simulink model "CSWI"  (Simulink 7.8)
settings: Solver=ode3  StartTime=0.0  StopTime=t_sim  FixedStep=1/6400  MaxStep=0.001  MinStep=0.000005  RelTol=1e-3
StopFcn:
  | ComtradeWrite5( RDRE1_UIabc, RDRE1_ANames, RDRE1_Dsignals, RDRE1_DNames, RDRE1_ADCscale, RDRE1_PromtFile, RDRE1_NumFile, RDRE1_FileFormat, RDRE1_TestNum);
  | clear RDRE1_UIabc RDRE1_ANames RDRE1_Dsignals RDRE1_DNames RDRE1_ADCscale  RDRE1_PromtFile RDRE1_NumFile RDRE1_FileFormat RDRE1_TestNum
values from neighbouring files (symbols this model uses):
  BlkTmms1 = 700    [CSWI_SG1.m]    (also in CSWI_SG2.m = 650; CSWI_SG3.m; CSWI_SG4.m; CSWI_SG5.m)
  BlkTmms2 = 800    [CSWI_SG1.m]    (also in CSWI_SG2.m = 750; CSWI_SG3.m; CSWI_SG4.m; CSWI_SG5.m)
  ClsTmms1 = 250    [CSWI_SG1.m]    (also in CSWI_SG2.m = 200; CSWI_SG3.m; CSWI_SG4.m; CSWI_SG5.m)
  ClsTmms2 = 170    [CSWI_SG1.m]    (also in CSWI_SG2.m = 100; CSWI_SG3.m; CSWI_SG4.m; CSWI_SG5.m)
  ClsTmms3 = 60    [CSWI_SG1.m]    (also in CSWI_SG2.m = 30; CSWI_SG3.m; CSWI_SG4.m; CSWI_SG5.m)
  ClsTmms4 = 10    [CSWI_SG1.m]    (also in CSWI_SG2.m = 20; CSWI_SG3.m; CSWI_SG4.m; CSWI_SG5.m)
  FailTmms = 350    [CSWI_SG1.m]    (also in CSWI_SG2.m = 300; CSWI_SG3.m; CSWI_SG4.m; CSWI_SG5.m)
  FctMod1 = 1    [CSWI_SG1.m]    (also in CSWI_SG2.m; CSWI_SG3.m; CSWI_SG4.m; CSWI_SG5.m)
  FctMod2 = 1    [CSWI_SG1.m]    (also in CSWI_SG2.m; CSWI_SG3.m; CSWI_SG4.m = 0; CSWI_SG5.m)
  FctMod3 = 1    [CSWI_SG1.m]    (also in CSWI_SG2.m; CSWI_SG3.m; CSWI_SG4.m; CSWI_SG5.m = 0)
  Num_SG = 1    [CSWI_generate_tests.m]
  OpnTmms1 = 300    [CSWI_SG1.m]    (also in CSWI_SG2.m = 250; CSWI_SG3.m; CSWI_SG4.m; CSWI_SG5.m)
  OpnTmms2 = 200    [CSWI_SG1.m]    (also in CSWI_SG2.m = 150; CSWI_SG3.m; CSWI_SG4.m; CSWI_SG5.m)
  OpnTmms3 = 30    [CSWI_SG1.m]    (also in CSWI_SG2.m = 90; CSWI_SG3.m = 90; CSWI_SG4.m; CSWI_SG5.m)
  test_dc = 'Ïðîâåðêà îòñóòñòâèÿ ôîðìèðîâàíèÿ ñèãíàëîâ "Âêë." ïðè ôîðìèðîâàíèè ñèãíàëà  "Îòêë. îò ÄÓ"'    [CSWI_generate_tests.m]
undefined symbols (not defined in the file or in its folder): sigbuilder_block, Test_num
libraries: powerlib_extras x21
(part 3 of 3)

== system CSWI/CSWI/Положение блок-контактов/BlkTmms1/ON Delay ==
  IN : Inport
  DELAY : Inport  Port=2
  Enable : EnablePort  PropagateVarSize=During execution
  Constant2 : Constant  Value=-Ts
  Constant3 : Constant  Value=Ts
  Discrete Edge Detector : powerlib_extras/Discrete  Control Blocks/Discrete Edge Detector  model=Rising  ic=ic  Ts=Ts
  Logical Operator1 : Logic
  Relational Operator : RelationalOperator  OutDataTypeStr=boolean  InputSameDT=on
  Sum1 : Sum  Inputs=+-  SaturateOnIntegerOverflow=on  InputSameDT=on  OutDataTypeStr=Inherit: Same as first input
  Switch : Switch  Threshold=0.5  SaturateOnIntegerOverflow=on  InputSameDT=on
  Unit Delay : UnitDelay  SampleTime=Ts
  OUT : Outport
  wires:
  Unit Delay/1 -> Switch/3
  Sum1/1 -> Unit Delay/1, Relational Operator/2
  Switch/1 -> Sum1/1
  Constant3/1 -> Sum1/2
  Relational Operator/1 -> Logical Operator1/2
  IN/1 -> Discrete Edge Detector/1, Logical Operator1/1
  Logical Operator1/1 -> OUT/1
  DELAY/1 -> Switch/1
  Discrete Edge Detector/1 -> Switch/2
  Constant2/1 -> Relational Operator/1

== system CSWI/CSWI/Положение блок-контактов/BlkTmms2/OFF Delay ==
  IN : Inport
  DELAY : Inport  Port=2
  Enable : EnablePort  PropagateVarSize=During execution
  Constant2 : Constant  Value=-Ts
  Constant3 : Constant  Value=Ts
  Discrete Edge Detector : powerlib_extras/Discrete  Control Blocks/Discrete Edge Detector  model=Falling  ic=ic  Ts=Ts
  Logical Operator1 : Logic
  Logical Operator2 : Logic  Operator=NOT
  Logical Operator3 : Logic  Operator=NOT
  Relational Operator : RelationalOperator  OutDataTypeStr=boolean  InputSameDT=on
  Sum1 : Sum  Inputs=+-  SaturateOnIntegerOverflow=on  InputSameDT=on  OutDataTypeStr=Inherit: Same as first input
  Switch : Switch  Threshold=0.5  SaturateOnIntegerOverflow=on  InputSameDT=on
  Unit Delay : UnitDelay  SampleTime=Ts
  OUT : Outport
  wires:
  Unit Delay/1 -> Switch/3
  Sum1/1 -> Relational Operator/2, Unit Delay/1
  Switch/1 -> Sum1/1
  Constant3/1 -> Sum1/2
  Relational Operator/1 -> Logical Operator1/2
  IN/1 -> Discrete Edge Detector/1, Logical Operator2/1
  Logical Operator1/1 -> Logical Operator3/1
  DELAY/1 -> Switch/1
  Discrete Edge Detector/1 -> Switch/2
  Constant2/1 -> Relational Operator/1
  Logical Operator2/1 -> Logical Operator1/1
  Logical Operator3/1 -> OUT/1

== system CSWI/CSWI/Положение блок-контактов/BlkTmms2/ON Delay ==
  IN : Inport
  DELAY : Inport  Port=2
  Enable : EnablePort  PropagateVarSize=During execution
  Constant2 : Constant  Value=-Ts
  Constant3 : Constant  Value=Ts
  Discrete Edge Detector : powerlib_extras/Discrete  Control Blocks/Discrete Edge Detector  model=Rising  ic=ic  Ts=Ts
  Logical Operator1 : Logic
  Relational Operator : RelationalOperator  OutDataTypeStr=boolean  InputSameDT=on
  Sum1 : Sum  Inputs=+-  SaturateOnIntegerOverflow=on  InputSameDT=on  OutDataTypeStr=Inherit: Same as first input
  Switch : Switch  Threshold=0.5  SaturateOnIntegerOverflow=on  InputSameDT=on
  Unit Delay : UnitDelay  SampleTime=Ts
  OUT : Outport
  wires:
  Unit Delay/1 -> Switch/3
  Sum1/1 -> Unit Delay/1, Relational Operator/2
  Switch/1 -> Sum1/1
  Constant3/1 -> Sum1/2
  Relational Operator/1 -> Logical Operator1/2
  IN/1 -> Discrete Edge Detector/1, Logical Operator1/1
  Logical Operator1/1 -> OUT/1
  DELAY/1 -> Switch/1
  Discrete Edge Detector/1 -> Switch/2
  Constant2/1 -> Relational Operator/1

== system CSWI/CSWI/Положение блок-контактов/BlkTmms3/OFF Delay ==
  IN : Inport
  DELAY : Inport  Port=2
  Enable : EnablePort  PropagateVarSize=During execution
  Constant2 : Constant  Value=-Ts
  Constant3 : Constant  Value=Ts
  Discrete Edge Detector : powerlib_extras/Discrete  Control Blocks/Discrete Edge Detector  model=Falling  ic=ic  Ts=Ts
  Logical Operator1 : Logic
  Logical Operator2 : Logic  Operator=NOT
  Logical Operator3 : Logic  Operator=NOT
  Relational Operator : RelationalOperator  OutDataTypeStr=boolean  InputSameDT=on
  Sum1 : Sum  Inputs=+-  SaturateOnIntegerOverflow=on  InputSameDT=on  OutDataTypeStr=Inherit: Same as first input
  Switch : Switch  Threshold=0.5  SaturateOnIntegerOverflow=on  InputSameDT=on
  Unit Delay : UnitDelay  SampleTime=Ts
  OUT : Outport
  wires:
  Unit Delay/1 -> Switch/3
  Sum1/1 -> Relational Operator/2, Unit Delay/1
  Switch/1 -> Sum1/1
  Constant3/1 -> Sum1/2
  Relational Operator/1 -> Logical Operator1/2
  IN/1 -> Discrete Edge Detector/1, Logical Operator2/1
  Logical Operator1/1 -> Logical Operator3/1
  DELAY/1 -> Switch/1
  Discrete Edge Detector/1 -> Switch/2
  Constant2/1 -> Relational Operator/1
  Logical Operator2/1 -> Logical Operator1/1
  Logical Operator3/1 -> OUT/1

== system CSWI/CSWI/Положение блок-контактов/BlkTmms3/ON Delay ==
  IN : Inport
  DELAY : Inport  Port=2
  Enable : EnablePort  PropagateVarSize=During execution
  Constant2 : Constant  Value=-Ts
  Constant3 : Constant  Value=Ts
  Discrete Edge Detector : powerlib_extras/Discrete  Control Blocks/Discrete Edge Detector  model=Rising  ic=ic  Ts=Ts
  Logical Operator1 : Logic
  Relational Operator : RelationalOperator  OutDataTypeStr=boolean  InputSameDT=on
  Sum1 : Sum  Inputs=+-  SaturateOnIntegerOverflow=on  InputSameDT=on  OutDataTypeStr=Inherit: Same as first input
  Switch : Switch  Threshold=0.5  SaturateOnIntegerOverflow=on  InputSameDT=on
  Unit Delay : UnitDelay  SampleTime=Ts
  OUT : Outport
  wires:
  Unit Delay/1 -> Switch/3
  Sum1/1 -> Unit Delay/1, Relational Operator/2
  Switch/1 -> Sum1/1
  Constant3/1 -> Sum1/2
  Relational Operator/1 -> Logical Operator1/2
  IN/1 -> Discrete Edge Detector/1, Logical Operator1/1
  Logical Operator1/1 -> OUT/1
  DELAY/1 -> Switch/1
  Discrete Edge Detector/1 -> Switch/2
  Constant2/1 -> Relational Operator/1

== system CSWI/CSWI/РФК и Аварийное отключение/Discrete Bistable7/RESET Priority ==
  S : Inport
  R : Inport  Port=2
  Enable : EnablePort  PropagateVarSize=During execution
  IC = ic : UnitDelay  X0=ic  SampleTime=Ts
  Logical Operator : Logic  Operator=OR
  Logical Operator1 : Logic  Operator=NOT  Inputs=1
  Logical Operator2 : Logic
  Logical Operator3 : Logic  Operator=NOT  Inputs=1
  Q : Outport
  !Q : Outport  Port=2
  wires:
  Logical Operator2/1 -> Q/1, Logical Operator3/1, IC = ic/1
  Logical Operator1/1 -> Logical Operator2/2
  R/1 -> Logical Operator1/1
  Logical Operator/1 -> Logical Operator2/1
  IC = ic/1 -> Logical Operator/2
  Logical Operator3/1 -> !Q/1
  S/1 -> Logical Operator/1

== system CSWI/CSWI/РФК и Аварийное отключение/Discrete Bistable7/SET  Priority ==
  S : Inport
  R : Inport  Port=2
  Enable : EnablePort  PropagateVarSize=During execution
  IC = ic : UnitDelay  X0=ic  SampleTime=Ts
  Logical Operator : Logic  Operator=OR
  Logical Operator1 : Logic  Operator=NOT  Inputs=1
  Logical Operator2 : Logic
  Logical Operator3 : Logic  Operator=NOT  Inputs=1
  Q : Outport
  !Q : Outport  Port=2
  wires:
  S/1 -> Logical Operator/1
  Logical Operator3/1 -> !Q/1
  Logical Operator/1 -> IC = ic/1, Logical Operator3/1, Q/1
  R/1 -> Logical Operator1/1
  Logical Operator1/1 -> Logical Operator2/1
  IC = ic/1 -> Logical Operator2/2
  Logical Operator2/1 -> Logical Operator/2

== system CSWI/CSWI/Блок включения/ClsTmms2/Edge_Detector/NEGATIVE Edge ==
  IN : Inport
  IN previous : Inport  Port=2
  Enable : EnablePort  PropagateVarSize=During execution
  Relational Operator1 : RelationalOperator  Operator=>  InputSameDT=on
  OUT : Outport
  wires:
  IN/1 -> Relational Operator1/2
  IN previous/1 -> Relational Operator1/1
  Relational Operator1/1 -> OUT/1

== system CSWI/CSWI/Блок включения/ClsTmms2/Edge_Detector/POSITIVE Edge ==
  IN : Inport
  IN previous : Inport  Port=2
  Enable : EnablePort  PropagateVarSize=During execution
  Relational Operator1 : RelationalOperator  Operator=>  InputSameDT=on
  OUT : Outport
  wires:
  IN/1 -> Relational Operator1/1
  IN previous/1 -> Relational Operator1/2
  Relational Operator1/1 -> OUT/1

== system CSWI/CSWI/Блок отключения/OpnTmms2/Edge_Detector/NEGATIVE Edge ==
  IN : Inport
  IN previous : Inport  Port=2
  Enable : EnablePort  PropagateVarSize=During execution
  Relational Operator1 : RelationalOperator  Operator=>  InputSameDT=on
  OUT : Outport
  wires:
  IN/1 -> Relational Operator1/2
  IN previous/1 -> Relational Operator1/1
  Relational Operator1/1 -> OUT/1

== system CSWI/CSWI/Блок отключения/OpnTmms2/Edge_Detector/POSITIVE Edge ==
  IN : Inport
  IN previous : Inport  Port=2
  Enable : EnablePort  PropagateVarSize=During execution
  Relational Operator1 : RelationalOperator  Operator=>  InputSameDT=on
  OUT : Outport
  wires:
  IN/1 -> Relational Operator1/1
  IN previous/1 -> Relational Operator1/2
  Relational Operator1/1 -> OUT/1

== matlab function DREGOUT1/MATLAB Function ==
  data: u input double; SG_1 output double; SG_2 output double; SG_3 output double; SG_4 output double; SG_5 output double; SG_6 output double
% function [SG_1,SG_2,SG_3,SG_4]= fcn(u)
function [SG_1,SG_2,SG_3,SG_4,SG_5,SG_6]= fcn(u)
%#codegen
SG_1=0; SG_2=0; SG_3=0; SG_4=0; SG_5=0; SG_6=0;


if u ==2;
    SG_1=1;
elseif u ==3;
    SG_2=1;
elseif u ==4;
    SG_1=1; SG_2=1;
elseif u ==5;
    SG_3=1;
elseif u ==6;
    SG_1=1; SG_3=1;
elseif u ==7;
    SG_2=1; SG_3=1;
elseif u ==8;
    SG_1=1; SG_2=1; SG_3=1;
elseif u ==9;
    SG_4=1;
elseif u ==10;
    SG_1=1; SG_4=1;
elseif u ==11;
    SG_2=1; SG_4=1;
elseif u ==12;
    SG_1=1; SG_2=1; SG_4=1;
elseif u ==13;
    SG_3=1; SG_4=1;
elseif u ==14;
    SG_1=1; SG_3=1; SG_4=1;
elseif u ==15;
    SG_2=1; SG_3=1; SG_4=1;
elseif u ==16;
    SG_1=1; SG_2=1; SG_3=1; SG_4=1;
elseif u ==17;
    SG_5=1;
    
elseif u ==18;
       SG_5=1; SG_1=1;  
elseif u ==19;
       SG_5=1; SG_2=1;     
elseif u ==20;
       SG_5=1; SG_2=1; SG_1=1; 
elseif u ==21;
       SG_5=1; SG_3=1; 
elseif u ==22;
       SG_5=1; SG_3=1; SG_1=1;
elseif u ==23;
       SG_5=1; SG_3=1; SG_2=1;
elseif u ==24;
       SG_5=1; SG_3=1; SG_2=1; SG_1=1;
elseif u ==25;
       SG_5=1; SG_4=1;
elseif u ==26;
       SG_5=1; SG_4=1; SG_1=1;
elseif u ==27;
       SG_5=1; SG_4=1; SG_2=1;
elseif u ==28;
       SG_5=1; SG_4=1; SG_2=1; SG_1=1;
elseif u ==29;
       SG_5=1; SG_4=1; SG_3=1;    
elseif u ==30;
       SG_5=1; SG_4=1; SG_3=1; SG_1=1;
elseif u ==31;
       SG_5=1; SG_4=1; SG_3=1; SG_2=1;
elseif u ==32;
       SG_5=1; SG_4=1; SG_3=1; SG_2=1; SG_1=1;
elseif u ==33;
       SG_6=1;
elseif u ==34;
       SG_6=1; SG_1=1;
elseif u ==35;
       SG_6=1; SG_2=1;
elseif u ==36;
       SG_6=1; SG_2=1; SG_1=1;
elseif u ==37;
       SG_6=1; SG_3=1;
elseif u ==38;
       SG_6=1; SG_3=1; SG_1=1;
elseif u ==39;
       SG_6=1; SG_3=1; SG_2=1;
elseif u ==40;
       SG_6=1; SG_3=1; SG_2=1; SG_1=1;   
elseif u ==41;
       SG_6=1; SG_4=1;    
elseif u ==42;
       SG_6=1; SG_4=1; SG_1=1;
elseif u ==43;
       SG_6=1; SG_4=1; SG_2=1;
elseif u ==44;
       SG_6=1; SG_4=1; SG_2=1; SG_1=1;
elseif u ==45;
       SG_6=1; SG_4=1; SG_3=1;
elseif u ==46;
       SG_6=1; SG_4=1; SG_3=1; SG_1=1;
elseif u ==47;
       SG_6=1; SG_4=1; SG_3=1; SG_2=1;
elseif u ==48;
       SG_6=1; SG_4=1; SG_3=1; SG_2=1; SG_1=1;
elseif u ==49;
       SG_6=1; SG_5=1;
elseif u ==50;
       SG_6=1; SG_5=1; SG_1=1;
elseif u ==51;
       SG_6=1; SG_5=1; SG_2=1;
elseif u ==52;
       SG_6=1; SG_5=1; SG_2=1; SG_1=1;
elseif u ==53;
       SG_6=1; SG_5=1; SG_3=1;
elseif u ==54;
       SG_6=1; SG_5=1; SG_3=1; SG_1=1;
elseif u ==55;
       SG_6=1; SG_5=1; SG_3=1; SG_2=1;
elseif u ==56;
       SG_6=1; SG_5=1; SG_3=1; SG_2=1; SG_1=1;
elseif u ==57;
       SG_6=1; SG_5=1; SG_4=1;
elseif u ==58;
       SG_6=1; SG_5=1; SG_4=1; SG_1=1;
elseif u ==59;
       SG_6=1; SG_5=1; SG_4=1; SG_2=1;
elseif u ==60;
       SG_6=1; SG_5=1; SG_4=1; SG_2=1; SG_1=1;
elseif u ==61;
       SG_6=1; SG_5=1; SG_4=1; SG_3=1;
elseif u ==62;
       SG_6=1; SG_5=1; SG_4=1; SG_3=1; SG_1=1;
elseif u ==63;
       SG_6=1; SG_5=1; SG_4=1; SG_3=1; SG_2=1;
elseif u ==64;
       SG_6=1; SG_5=1; SG_4=1; SG_3=1; SG_2=1; SG_1=1;
    
end
% bincode = dec2bin (u-1);

% if size (bincode,2) == 1
%    SG_1 = str2double(bincode(1,1));
% end
% 
% if size (bincode,2) == 2
%    SG_1 = str2double(bincode(1,1));
%    SG_2 = str2double(bincode(1,2));
% end
% 
% if size (bincode,2) == 3
%    SG_1 = str2double(bincode(1,1));
%    SG_2 = str2double(bincode(1,2));
%    SG_3 = str2double(bincode(1,3));
% end
% 
% if size (bincode,2) == 4
%    SG_1 = str2double(bincode(1,1));
%    SG_2 = str2double(bincode(1,2));
%    SG_3 = str2double(bincode(1,3));
%    SG_4 = str2double(bincode(1,4));
% end
% 
% end
